simulink library "IPT_FCM_lib"  (Simulink 7.4)
settings: Solver=ode45  StartTime=0.0  StopTime=10.0  RelTol=1e-3
libraries: Defined_Functionality x62
settings Model: Creator=sunsijun  LastModifiedBy=sunsijun

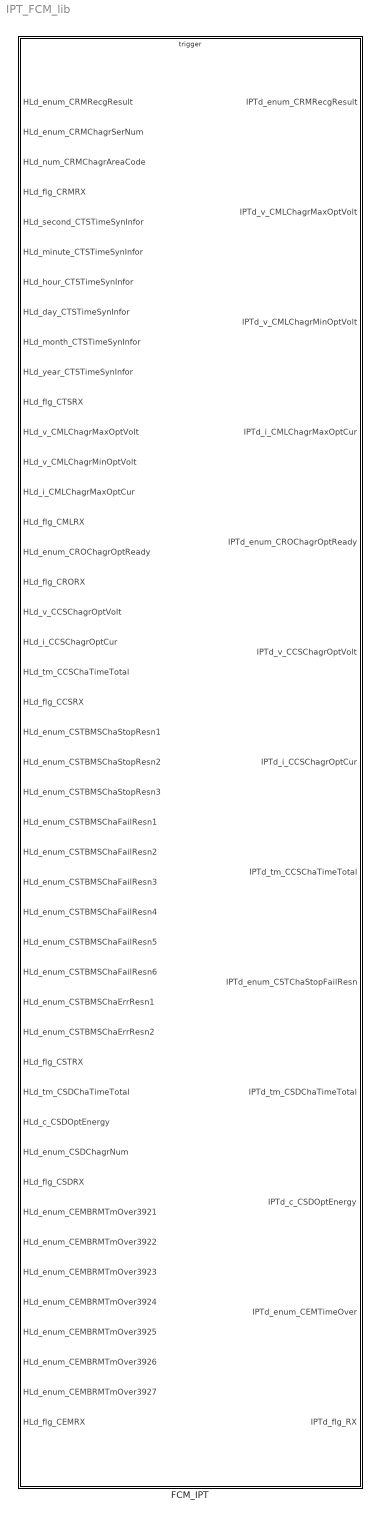
== system IPT_FCM_lib ==
  FCM_IPT : Subsystem  TreatAsAtomicUnit=on
      settings: RTWSystemCode=Function  RTWFcnNameOpts=Use subsystem name

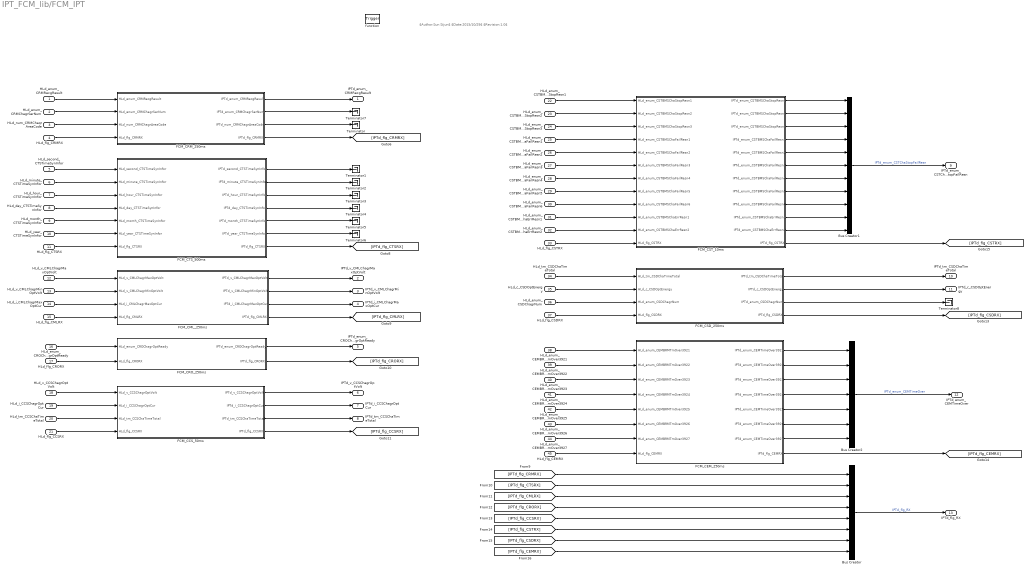
== system IPT_FCM_lib/FCM_IPT ==
  note: $Author:Sun Sijun$
      | $Date:2015/10/29$
      | $Revision:1.0$
  HLd_enum_CRMRecgResult : Inport
  HLd_enum_CRMChagrSerNum : Inport  Port=2
  HLd_num_CRMChagrAreaCode : Inport  Port=3
  HLd_flg_CRMRX : Inport  Port=4
  HLd_second_CTSTimeSynInfor : Inport  Port=5
  HLd_minute_CTSTimeSynInfor : Inport  Port=6
  HLd_hour_CTSTimeSynInfor : Inport  Port=7
  HLd_day_CTSTimeSynInfor : Inport  Port=8
  HLd_month_CTSTimeSynInfor : Inport  Port=9
  HLd_year_CTSTimeSynInfor : Inport  Port=10
  HLd_flg_CTSRX : Inport  Port=11
  HLd_v_CMLChagrMaxOptVolt : Inport  Port=12
  HLd_v_CMLChagrMinOptVolt : Inport  Port=13
  HLd_i_CMLChagrMaxOptCur : Inport  Port=14
  HLd_flg_CMLRX : Inport  Port=15
  HLd_enum_CROChagrOptReady : Inport  Port=16
  HLd_flg_CRORX : Inport  Port=17
  HLd_v_CCSChagrOptVolt : Inport  Port=18
  HLd_i_CCSChagrOptCur : Inport  Port=19
  HLd_tm_CCSChaTimeTotal : Inport  Port=20
  HLd_flg_CCSRX : Inport  Port=21
  HLd_enum_CSTBMSChaStopResn1 : Inport  Port=22
  HLd_enum_CSTBMSChaStopResn2 : Inport  Port=23
  HLd_enum_CSTBMSChaStopResn3 : Inport  Port=24
  HLd_enum_CSTBMSChaFailResn1 : Inport  Port=25
  HLd_enum_CSTBMSChaFailResn2 : Inport  Port=26
  HLd_enum_CSTBMSChaFailResn3 : Inport  Port=27
  HLd_enum_CSTBMSChaFailResn4 : Inport  Port=28
  HLd_enum_CSTBMSChaFailResn5 : Inport  Port=29
  HLd_enum_CSTBMSChaFailResn6 : Inport  Port=30
  HLd_enum_CSTBMSChaErrResn1 : Inport  Port=31
  HLd_enum_CSTBMSChaErrResn2 : Inport  Port=32
  HLd_flg_CSTRX : Inport  Port=33
  HLd_tm_CSDChaTimeTotal : Inport  Port=34
  HLd_c_CSDOptEnergy : Inport  Port=35
  HLd_enum_CSDChagrNum : Inport  Port=36
  HLd_flg_CSDRX : Inport  Port=37
  HLd_enum_CEMBRMTmOver3921 : Inport  Port=38
  HLd_enum_CEMBRMTmOver3922 : Inport  Port=39
  HLd_enum_CEMBRMTmOver3923 : Inport  Port=40
  HLd_enum_CEMBRMTmOver3924 : Inport  Port=41
  HLd_enum_CEMBRMTmOver3925 : Inport  Port=42
  HLd_enum_CEMBRMTmOver3926 : Inport  Port=43
  HLd_enum_CEMBRMTmOver3927 : Inport  Port=44
  HLd_flg_CEMRX : Inport  Port=45
  function : TriggerPort  TriggerType=function-call
  Bus Creator : BusCreator  Inputs=8
  Bus Creator1 : BusCreator  Inputs=11
  Bus Creator2 : BusCreator  Inputs=7
  FCM_CCS_50ms : Subsystem
      settings: RTWFcnNameOpts=Use subsystem name  RTWFileNameOpts=Use subsystem name
  FCM_CEM_250ms : Subsystem
      settings: RTWFcnNameOpts=Use subsystem name  RTWFileNameOpts=Use subsystem name
  FCM_CML_250ms : Subsystem
      settings: RTWFcnNameOpts=Use subsystem name  RTWFileNameOpts=Use subsystem name
  FCM_CRM_250ms : Subsystem
      settings: RTWFcnNameOpts=Use subsystem name  RTWFileNameOpts=Use subsystem name
  FCM_CRO_250ms : Subsystem
      settings: RTWFcnNameOpts=Use subsystem name  RTWFileNameOpts=Use subsystem name
  FCM_CSD_250ms : Subsystem
      settings: RTWFcnNameOpts=Use subsystem name  RTWFileNameOpts=Use subsystem name
  FCM_CST_10ms : Subsystem
      settings: RTWFcnNameOpts=Use subsystem name  RTWFileNameOpts=Use subsystem name
  FCM_CTS_500ms : Subsystem
      settings: RTWFcnNameOpts=Use subsystem name  RTWFileNameOpts=Use subsystem name
  Terminator{,1..8} (9 alike) : Terminator
  IPTd_enum_CRMRecgResult : Outport
  IPTd_v_CMLChagrMaxOptVolt : Outport  Port=2
  IPTd_v_CMLChagrMinOptVolt : Outport  Port=3
  IPTd_i_CMLChagrMaxOptCur : Outport  Port=4
  IPTd_enum_CROChagrOptReady : Outport  Port=5
  IPTd_v_CCSChagrOptVolt : Outport  Port=6
  IPTd_i_CCSChagrOptCur : Outport  Port=7
  IPTd_tm_CCSChaTimeTotal : Outport  Port=8
  IPTd_enum_CSTChaStopFailResn : Outport  Port=9
  IPTd_tm_CSDChaTimeTotal : Outport  Port=10
  IPTd_c_CSDOptEnergy : Outport  Port=11
  IPTd_enum_CEMTimeOver : Outport  Port=12
  IPTd_flg_RX : Outport  Port=13
  wires:
  HLd_flg_CEMRX/1 -> FCM_CEM_250ms/8(HLd_flg_CEMRX)
  HLd_flg_CSDRX/1 -> FCM_CSD_250ms/4(HLd_flg_CSDRX)
  HLd_flg_CSTRX/1 -> FCM_CST_10ms/12(HLd_flg_CSTRX)
  HLd_flg_CCSRX/1 -> FCM_CCS_50ms/4(HLd_flg_CCSRX)
  HLd_flg_CRORX/1 -> FCM_CRO_250ms/2(HLd_flg_CRORX)
  HLd_flg_CMLRX/1 -> FCM_CML_250ms/4(HLd_flg_CMLRX)
  HLd_flg_CTSRX/1 -> FCM_CTS_500ms/7(HLd_flg_CTSRX)
  HLd_flg_CRMRX/1 -> FCM_CRM_250ms/4(HLd_flg_CRMRX)
  Bus Creator1/1 -> IPTd_enum_CSTChaStopFailResn/1  "IPTd_enum_CSTChaStopFailResn"
  Bus Creator2/1 -> IPTd_enum_CEMTimeOver/1  "IPTd_enum_CEMTimeOver"
  FCM_CST_10ms/11(IPTd_enum_CSTBMSChaErrResn2) -> Bus Creator1/11
  FCM_CST_10ms/10(IPTd_enum_CSTBMSChaErrResn1) -> Bus Creator1/10
  FCM_CST_10ms/9(IPTd_enum_CSTBMSChaFailResn6) -> Bus Creator1/9
  FCM_CST_10ms/8(IPTd_enum_CSTBMSChaFailResn5) -> Bus Creator1/8
  FCM_CST_10ms/7(IPTd_enum_CSTBMSChaFailResn4) -> Bus Creator1/7
  FCM_CST_10ms/6(IPTd_enum_CSTBMSChaFailResn3) -> Bus Creator1/6
  FCM_CST_10ms/5(IPTd_enum_CSTBMSChaFailResn2) -> Bus Creator1/5
  FCM_CST_10ms/4(IPTd_enum_CSTBMSChaFailResn1) -> Bus Creator1/4
  FCM_CST_10ms/3(IPTd_enum_CSTBMSChaStopResn3) -> Bus Creator1/3
  FCM_CST_10ms/2(IPTd_enum_CSTBMSChaStopResn2) -> Bus Creator1/2
  FCM_CST_10ms/1(IPTd_enum_CSTBMSChaStopResn1) -> Bus Creator1/1
  Bus Creator/1 -> IPTd_flg_RX/1  "IPTd_flg_RX"
  [IPTd_flg_CEMRX] -> Bus Creator/8
  [IPTd_flg_CSDRX] -> Bus Creator/7
  [IPTd_flg_CSTRX] -> Bus Creator/6
  [IPTd_flg_CCSRX] -> Bus Creator/5
  [IPTd_flg_CRORX] -> Bus Creator/4
  [IPTd_flg_CMLRX] -> Bus Creator/3
  [IPTd_flg_CTSRX] -> Bus Creator/2
  [IPTd_flg_CRMRX] -> Bus Creator/1
  FCM_CEM_250ms/8(IPTd_flg_CEMRX) -> [IPTd_flg_CEMRX]
  FCM_CSD_250ms/4(IPTd_flg_CSDRX) -> [IPTd_flg_CSDRX]
  FCM_CST_10ms/12(IPTd_flg_CSTRX) -> [IPTd_flg_CSTRX]
  FCM_CCS_50ms/4(IPTd_flg_CCSRX) -> [IPTd_flg_CCSRX]
  FCM_CRO_250ms/2(IPTd_flg_CRORX) -> [IPTd_flg_CRORX]
  FCM_CEM_250ms/1(IPTd_enum_CEMTimeOver3921) -> Bus Creator2/1
  FCM_CEM_250ms/2(IPTd_enum_CEMTimeOver3922) -> Bus Creator2/2
  FCM_CEM_250ms/3(IPTd_enum_CEMTimeOver3923) -> Bus Creator2/3
  FCM_CEM_250ms/4(IPTd_enum_CEMTimeOver3924) -> Bus Creator2/4
  FCM_CEM_250ms/5(IPTd_enum_CEMTimeOver3925) -> Bus Creator2/5
  FCM_CEM_250ms/6(IPTd_enum_CEMTimeOver3926) -> Bus Creator2/6
  FCM_CEM_250ms/7(IPTd_enum_CEMTimeOver3927) -> Bus Creator2/7
  HLd_enum_CEMBRMTmOver3921/1 -> FCM_CEM_250ms/1(HLd_enum_CEMBRMTmOver3921)
  HLd_enum_CEMBRMTmOver3922/1 -> FCM_CEM_250ms/2(HLd_enum_CEMBRMTmOver3922)
  HLd_enum_CEMBRMTmOver3923/1 -> FCM_CEM_250ms/3(HLd_enum_CEMBRMTmOver3923)
  HLd_enum_CEMBRMTmOver3924/1 -> FCM_CEM_250ms/4(HLd_enum_CEMBRMTmOver3924)
  HLd_enum_CEMBRMTmOver3925/1 -> FCM_CEM_250ms/5(HLd_enum_CEMBRMTmOver3925)
  HLd_enum_CEMBRMTmOver3926/1 -> FCM_CEM_250ms/6(HLd_enum_CEMBRMTmOver3926)
  HLd_enum_CEMBRMTmOver3927/1 -> FCM_CEM_250ms/7(HLd_enum_CEMBRMTmOver3927)
  HLd_tm_CSDChaTimeTotal/1 -> FCM_CSD_250ms/1(HLd_tm_CSDChaTimeTotal)
  HLd_c_CSDOptEnergy/1 -> FCM_CSD_250ms/2(HLd_c_CSDOptEnergy)
  HLd_enum_CSDChagrNum/1 -> FCM_CSD_250ms/3(HLd_enum_CSDChagrNum)
  FCM_CSD_250ms/3(IPTd_enum_CSDChagrNum) -> Terminator8/1
  FCM_CSD_250ms/2(IPTd_c_CSDOptEnergy) -> IPTd_c_CSDOptEnergy/1
  FCM_CSD_250ms/1(IPTd_tm_CSDChaTimeTotal) -> IPTd_tm_CSDChaTimeTotal/1
  HLd_enum_CSTBMSChaErrResn2/1 -> FCM_CST_10ms/11(HLd_enum_CSTBMSChaErrResn2)
  HLd_enum_CSTBMSChaErrResn1/1 -> FCM_CST_10ms/10(HLd_enum_CSTBMSChaErrResn1)
  HLd_enum_CSTBMSChaFailResn6/1 -> FCM_CST_10ms/9(HLd_enum_CSTBMSChaFailResn6)
  HLd_enum_CSTBMSChaFailResn5/1 -> FCM_CST_10ms/8(HLd_enum_CSTBMSChaFailResn5)
  HLd_enum_CSTBMSChaFailResn4/1 -> FCM_CST_10ms/7(HLd_enum_CSTBMSChaFailResn4)
  HLd_enum_CSTBMSChaFailResn3/1 -> FCM_CST_10ms/6(HLd_enum_CSTBMSChaFailResn3)
  HLd_enum_CSTBMSChaFailResn2/1 -> FCM_CST_10ms/5(HLd_enum_CSTBMSChaFailResn2)
  HLd_enum_CSTBMSChaFailResn1/1 -> FCM_CST_10ms/4(HLd_enum_CSTBMSChaFailResn1)
  HLd_enum_CSTBMSChaStopResn3/1 -> FCM_CST_10ms/3(HLd_enum_CSTBMSChaStopResn3)
  HLd_enum_CSTBMSChaStopResn2/1 -> FCM_CST_10ms/2(HLd_enum_CSTBMSChaStopResn2)
  HLd_enum_CSTBMSChaStopResn1/1 -> FCM_CST_10ms/1(HLd_enum_CSTBMSChaStopResn1)
  FCM_CCS_50ms/3(IPTd_tm_CCSChaTimeTotal) -> IPTd_tm_CCSChaTimeTotal/1
  FCM_CCS_50ms/2(IPTd_i_CCSChagrOptCur) -> IPTd_i_CCSChagrOptCur/1
  FCM_CCS_50ms/1(IPTd_v_CCSChagrOptVolt) -> IPTd_v_CCSChagrOptVolt/1
  HLd_tm_CCSChaTimeTotal/1 -> FCM_CCS_50ms/3(HLd_tm_CCSChaTimeTotal)
  HLd_i_CCSChagrOptCur/1 -> FCM_CCS_50ms/2(HLd_i_CCSChagrOptCur)
  HLd_v_CCSChagrOptVolt/1 -> FCM_CCS_50ms/1(HLd_v_CCSChagrOptVolt)
  HLd_enum_CROChagrOptReady/1 -> FCM_CRO_250ms/1(HLd_enum_CROChagrOptReady)
  FCM_CRO_250ms/1(IPTd_enum_CROChagrOptReady) -> IPTd_enum_CROChagrOptReady/1
  FCM_CML_250ms/1(IPTd_v_CMLChagrMaxOptVolt) -> IPTd_v_CMLChagrMaxOptVolt/1
  FCM_CML_250ms/2(IPTd_v_CMLChagrMinOptVolt) -> IPTd_v_CMLChagrMinOptVolt/1
  FCM_CML_250ms/3(IPTd_i_CMLChagrMaxOptCur) -> IPTd_i_CMLChagrMaxOptCur/1
  HLd_v_CMLChagrMaxOptVolt/1 -> FCM_CML_250ms/1(HLd_v_CMLChagrMaxOptVolt)
  HLd_v_CMLChagrMinOptVolt/1 -> FCM_CML_250ms/2(HLd_v_CMLChagrMinOptVolt)
  HLd_i_CMLChagrMaxOptCur/1 -> FCM_CML_250ms/3(HLd_i_CMLChagrMaxOptCur)
  HLd_year_CTSTimeSynInfor/1 -> FCM_CTS_500ms/6(HLd_year_CTSTimeSynInfor)
  HLd_month_CTSTimeSynInfor/1 -> FCM_CTS_500ms/5(HLd_month_CTSTimeSynInfor)
  HLd_day_CTSTimeSynInfor/1 -> FCM_CTS_500ms/4(HLd_day_CTSTimeSynInfor)
  HLd_hour_CTSTimeSynInfor/1 -> FCM_CTS_500ms/3(HLd_hour_CTSTimeSynInfor)
  HLd_minute_CTSTimeSynInfor/1 -> FCM_CTS_500ms/2(HLd_minute_CTSTimeSynInfor)
  HLd_second_CTSTimeSynInfor/1 -> FCM_CTS_500ms/1(HLd_second_CTSTimeSynInfor)
  FCM_CRM_250ms/3(IPTd_num_CRMChagrAreaCode) -> Terminator/1
  FCM_CRM_250ms/2(IPTd_enum_CRMChagrSerNum) -> Terminator7/1
  FCM_CRM_250ms/1(IPTd_enum_CRMRecgResult) -> IPTd_enum_CRMRecgResult/1
  HLd_num_CRMChagrAreaCode/1 -> FCM_CRM_250ms/3(HLd_num_CRMChagrAreaCode)
  HLd_enum_CRMChagrSerNum/1 -> FCM_CRM_250ms/2(HLd_enum_CRMChagrSerNum)
  HLd_enum_CRMRecgResult/1 -> FCM_CRM_250ms/1(HLd_enum_CRMRecgResult)
  FCM_CML_250ms/4(IPTd_flg_CMLRX) -> [IPTd_flg_CMLRX]
  FCM_CTS_500ms/6(IPTd_year_CTSTimeSynInfor) -> Terminator6/1
  FCM_CTS_500ms/5(IPTd_month_CTSTimeSynInfor) -> Terminator5/1
  FCM_CTS_500ms/4(IPTd_day_CTSTimeSynInfor) -> Terminator4/1
  FCM_CTS_500ms/3(IPTd_hour_CTSTimeSynInfor) -> Terminator3/1
  FCM_CTS_500ms/2(IPTd_minute_CTSTimeSynInfor) -> Terminator2/1
  FCM_CTS_500ms/1(IPTd_second_CTSTimeSynInfor) -> Terminator1/1
  FCM_CTS_500ms/7(IPTd_flg_CTSRX) -> [IPTd_flg_CTSRX]
  FCM_CRM_250ms/4(IPTd_flg_CRMRX) -> [IPTd_flg_CRMRX]

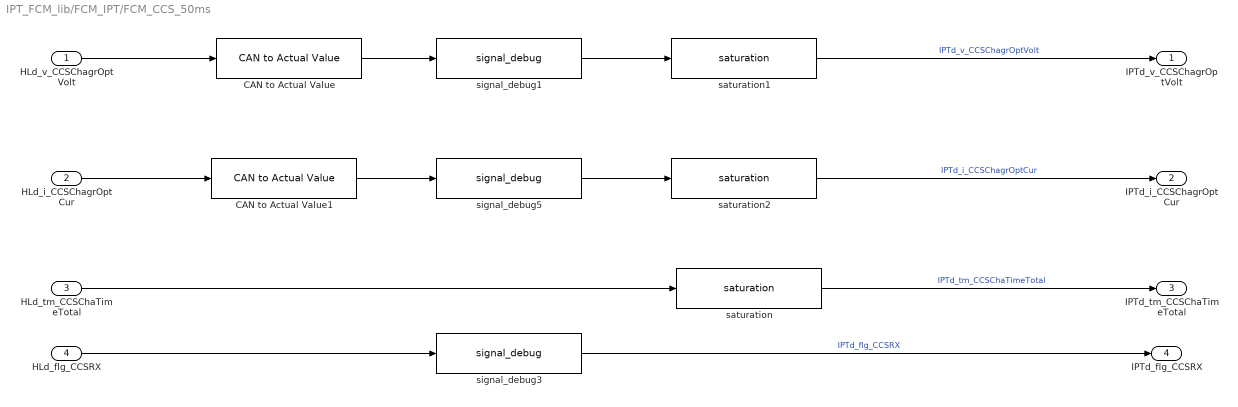
== system IPT_FCM_lib/FCM_IPT/FCM_CCS_50ms ==
  HLd_v_CCSChagrOptVolt : Inport
  HLd_i_CCSChagrOptCur : Inport  Port=2
  HLd_tm_CCSChaTimeTotal : Inport  Port=3
  HLd_flg_CCSRX : Inport  Port=4
  CAN to Actual Value : Defined_Functionality/CAN to Actual Value  SystemSampleTime=-1  gain=0.1  offset=0
      settings: AttributesFormatString=[GAIN=%<gain>]\n[OFFSET=%<offset>]
  CAN to Actual Value1 : Defined_Functionality/CAN to Actual Value  SystemSampleTime=-1  gain=0.1  offset=-400
      settings: AttributesFormatString=[GAIN=%<gain>]\n[OFFSET=%<offset>]
  saturation : Defined_Functionality/saturation  SystemSampleTime=-1  upper_limit=600  lower_limit=0
      settings: AttributesFormatString=[UPPER_LIMIT=%<upper_limit>]\n[LOWER_LIMIT=%<lower_limit>]
  saturation1 : Defined_Functionality/saturation  SystemSampleTime=-1  upper_limit=750  lower_limit=0
      settings: AttributesFormatString=[UPPER_LIMIT=%<upper_limit>]\n[LOWER_LIMIT=%<lower_limit>]
  saturation2 : Defined_Functionality/saturation  SystemSampleTime=-1  upper_limit=0  lower_limit=-400
      settings: AttributesFormatString=[UPPER_LIMIT=%<upper_limit>]\n[LOWER_LIMIT=%<lower_limit>]
  signal_debug1 : Defined_Functionality/signal_debug  SystemSampleTime=-1  debug_switch=IPTc_dbgsw_CCSChagrOptVolt  debug_value=IPTc_dbgval_CCSChagrOptVolt
      settings: AttributesFormatString=[SWITCH=%<debug_switch>]\n[VALUE=%<debug_value>]
  signal_debug3 : Defined_Functionality/signal_debug  SystemSampleTime=-1  debug_switch=IPTc_dbgsw_CCSRX  debug_value=IPTc_dbgval_CCSRX
      settings: AttributesFormatString=[SWITCH=%<debug_switch>]\n[VALUE=%<debug_value>]
  signal_debug5 : Defined_Functionality/signal_debug  SystemSampleTime=-1  debug_switch=IPTc_dbgsw_CCSChagrOptCur  debug_value=IPTc_dbgval_CCSChagrOptCur
      settings: AttributesFormatString=[SWITCH=%<debug_switch>]\n[VALUE=%<debug_value>]
  IPTd_v_CCSChagrOptVolt : Outport
  IPTd_i_CCSChagrOptCur : Outport  Port=2
  IPTd_tm_CCSChaTimeTotal : Outport  Port=3
  IPTd_flg_CCSRX : Outport  Port=4
  wires:
  HLd_flg_CCSRX/1 -> signal_debug3/1
  signal_debug3/1 -> IPTd_flg_CCSRX/1  "IPTd_flg_CCSRX"
  saturation2/1 -> IPTd_i_CCSChagrOptCur/1  "IPTd_i_CCSChagrOptCur"
  saturation1/1 -> IPTd_v_CCSChagrOptVolt/1  "IPTd_v_CCSChagrOptVolt"
  HLd_i_CCSChagrOptCur/1 -> CAN to Actual Value1/1
  HLd_v_CCSChagrOptVolt/1 -> CAN to Actual Value/1
  signal_debug1/1 -> saturation1/1
  CAN to Actual Value1/1 -> signal_debug5/1
  CAN to Actual Value/1 -> signal_debug1/1
  signal_debug5/1 -> saturation2/1
  saturation/1 -> IPTd_tm_CCSChaTimeTotal/1  "IPTd_tm_CCSChaTimeTotal"
  HLd_tm_CCSChaTimeTotal/1 -> saturation/1

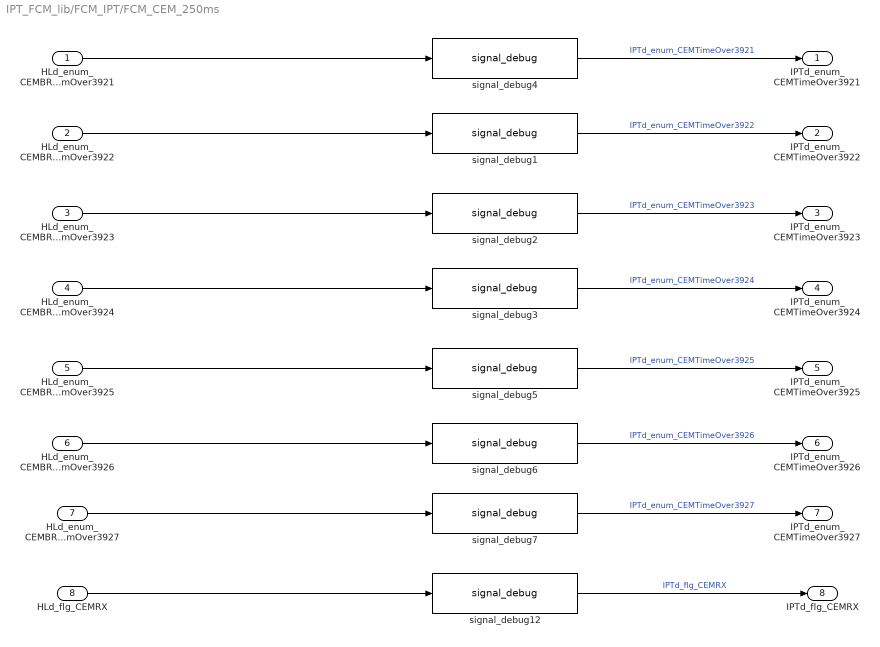
== system IPT_FCM_lib/FCM_IPT/FCM_CEM_250ms ==
  HLd_enum_CEMBRMTmOver3921 : Inport
  HLd_enum_CEMBRMTmOver3922 : Inport  Port=2
  HLd_enum_CEMBRMTmOver3923 : Inport  Port=3
  HLd_enum_CEMBRMTmOver3924 : Inport  Port=4
  HLd_enum_CEMBRMTmOver3925 : Inport  Port=5
  HLd_enum_CEMBRMTmOver3926 : Inport  Port=6
  HLd_enum_CEMBRMTmOver3927 : Inport  Port=7
  HLd_flg_CEMRX : Inport  Port=8
  signal_debug1 : Defined_Functionality/signal_debug  SystemSampleTime=-1  debug_switch=IPTc_dbgsw_CEMBRMTmOver3922  debug_value=IPTc_dbgval_CEMBRMTmOver3922
      settings: AttributesFormatString=[SWITCH=%<debug_switch>]\n[VALUE=%<debug_value>]
  signal_debug12 : Defined_Functionality/signal_debug  SystemSampleTime=-1  debug_switch=IPTc_dbgsw_CSDRX  debug_value=IPTc_dbgval_CSDRX
      settings: AttributesFormatString=[SWITCH=%<debug_switch>]\n[VALUE=%<debug_value>]
  signal_debug2 : Defined_Functionality/signal_debug  SystemSampleTime=-1  debug_switch=IPTc_dbgsw_CEMBRMTmOver3923  debug_value=IPTc_dbgval_CEMBRMTmOver3923
      settings: AttributesFormatString=[SWITCH=%<debug_switch>]\n[VALUE=%<debug_value>]
  signal_debug3 : Defined_Functionality/signal_debug  SystemSampleTime=-1  debug_switch=IPTc_dbgsw_CEMBRMTmOver3924  debug_value=IPTc_dbgval_CEMBRMTmOver3924
      settings: AttributesFormatString=[SWITCH=%<debug_switch>]\n[VALUE=%<debug_value>]
  signal_debug4 : Defined_Functionality/signal_debug  SystemSampleTime=-1  debug_switch=IPTc_dbgsw_CEMBRMTmOver3921  debug_value=IPTc_dbgval_CEMBRMTmOver3921
      settings: AttributesFormatString=[SWITCH=%<debug_switch>]\n[VALUE=%<debug_value>]
  signal_debug5 : Defined_Functionality/signal_debug  SystemSampleTime=-1  debug_switch=IPTc_dbgsw_CEMBRMTmOver3925  debug_value=IPTc_dbgval_CEMBRMTmOver3925
      settings: AttributesFormatString=[SWITCH=%<debug_switch>]\n[VALUE=%<debug_value>]
  signal_debug6 : Defined_Functionality/signal_debug  SystemSampleTime=-1  debug_switch=IPTc_dbgsw_CEMBRMTmOver3926  debug_value=IPTc_dbgval_CEMBRMTmOver3926
      settings: AttributesFormatString=[SWITCH=%<debug_switch>]\n[VALUE=%<debug_value>]
  signal_debug7 : Defined_Functionality/signal_debug  SystemSampleTime=-1  debug_switch=IPTc_dbgsw_CEMBRMTmOver3927  debug_value=IPTc_dbgval_CEMBRMTmOver3927
      settings: AttributesFormatString=[SWITCH=%<debug_switch>]\n[VALUE=%<debug_value>]
  IPTd_enum_CEMTimeOver3921 : Outport
  IPTd_enum_CEMTimeOver3922 : Outport  Port=2
  IPTd_enum_CEMTimeOver3923 : Outport  Port=3
  IPTd_enum_CEMTimeOver3924 : Outport  Port=4
  IPTd_enum_CEMTimeOver3925 : Outport  Port=5
  IPTd_enum_CEMTimeOver3926 : Outport  Port=6
  IPTd_enum_CEMTimeOver3927 : Outport  Port=7
  IPTd_flg_CEMRX : Outport  Port=8
  wires:
  signal_debug12/1 -> IPTd_flg_CEMRX/1  "IPTd_flg_CEMRX"
  HLd_flg_CEMRX/1 -> signal_debug12/1
  signal_debug5/1 -> IPTd_enum_CEMTimeOver3925/1  "IPTd_enum_CEMTimeOver3925"
  signal_debug7/1 -> IPTd_enum_CEMTimeOver3927/1  "IPTd_enum_CEMTimeOver3927"
  signal_debug6/1 -> IPTd_enum_CEMTimeOver3926/1  "IPTd_enum_CEMTimeOver3926"
  HLd_enum_CEMBRMTmOver3927/1 -> signal_debug7/1
  HLd_enum_CEMBRMTmOver3926/1 -> signal_debug6/1
  HLd_enum_CEMBRMTmOver3925/1 -> signal_debug5/1
  HLd_enum_CEMBRMTmOver3924/1 -> signal_debug3/1
  signal_debug3/1 -> IPTd_enum_CEMTimeOver3924/1  "IPTd_enum_CEMTimeOver3924"
  signal_debug2/1 -> IPTd_enum_CEMTimeOver3923/1  "IPTd_enum_CEMTimeOver3923"
  HLd_enum_CEMBRMTmOver3923/1 -> signal_debug2/1
  signal_debug1/1 -> IPTd_enum_CEMTimeOver3922/1  "IPTd_enum_CEMTimeOver3922"
  HLd_enum_CEMBRMTmOver3922/1 -> signal_debug1/1
  signal_debug4/1 -> IPTd_enum_CEMTimeOver3921/1  "IPTd_enum_CEMTimeOver3921"
  HLd_enum_CEMBRMTmOver3921/1 -> signal_debug4/1

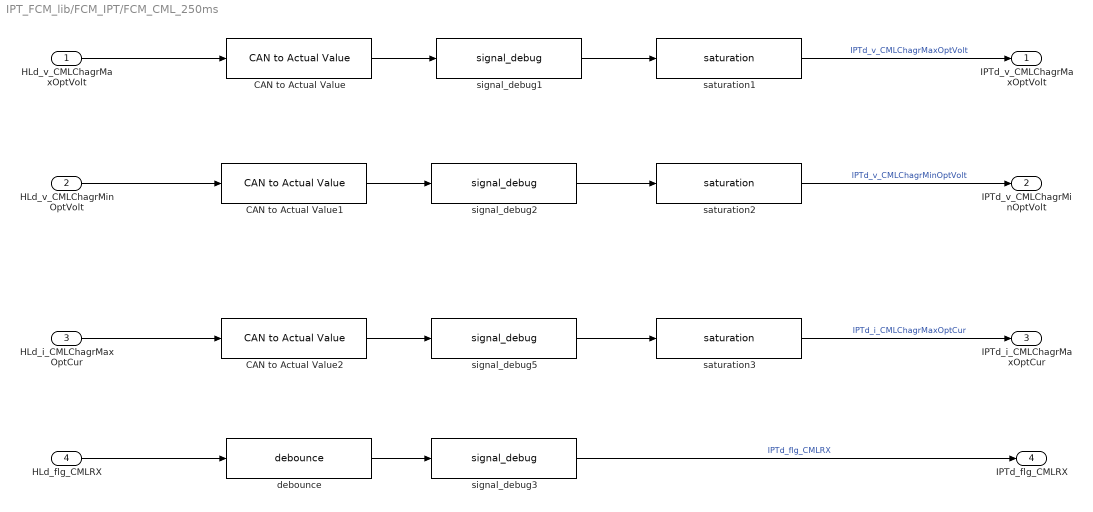
== system IPT_FCM_lib/FCM_IPT/FCM_CML_250ms ==
  HLd_v_CMLChagrMaxOptVolt : Inport
  HLd_v_CMLChagrMinOptVolt : Inport  Port=2
  HLd_i_CMLChagrMaxOptCur : Inport  Port=3
  HLd_flg_CMLRX : Inport  Port=4
  CAN to Actual Value : Defined_Functionality/CAN to Actual Value  SystemSampleTime=-1  gain=0.1  offset=0
      settings: AttributesFormatString=[GAIN=%<gain>]\n[OFFSET=%<offset>]
  CAN to Actual Value1 : Defined_Functionality/CAN to Actual Value  SystemSampleTime=-1  gain=0.1  offset=0
      settings: AttributesFormatString=[GAIN=%<gain>]\n[OFFSET=%<offset>]
  CAN to Actual Value2 : Defined_Functionality/CAN to Actual Value  SystemSampleTime=-1  gain=0.1  offset=-400
      settings: AttributesFormatString=[GAIN=%<gain>]\n[OFFSET=%<offset>]
  debounce : Defined_Functionality/debounce  SystemSampleTime=-1  debounce_time=30
      settings: AttributesFormatString=[DEBOUNCE_TIME=%<debounce_time>]
  saturation1 : Defined_Functionality/saturation  SystemSampleTime=-1  upper_limit=750  lower_limit=0
      settings: AttributesFormatString=[UPPER_LIMIT=%<upper_limit>]\n[LOWER_LIMIT=%<lower_limit>]
  saturation2 : Defined_Functionality/saturation  SystemSampleTime=-1  upper_limit=750  lower_limit=0
      settings: AttributesFormatString=[UPPER_LIMIT=%<upper_limit>]\n[LOWER_LIMIT=%<lower_limit>]
  saturation3 : Defined_Functionality/saturation  SystemSampleTime=-1  upper_limit=0  lower_limit=-400
      settings: AttributesFormatString=[UPPER_LIMIT=%<upper_limit>]\n[LOWER_LIMIT=%<lower_limit>]
  signal_debug1 : Defined_Functionality/signal_debug  SystemSampleTime=-1  debug_switch=IPTc_dbgsw_CMLChagrMaxOptVolt  debug_value=IPTc_dbgval_CMLChagrMaxOptVolt
      settings: AttributesFormatString=[SWITCH=%<debug_switch>]\n[VALUE=%<debug_value>]
  signal_debug2 : Defined_Functionality/signal_debug  SystemSampleTime=-1  debug_switch=IPTc_dbgsw_CMLChagrMinOptVolt  debug_value=IPTc_dbgval_CMLChagrMinOptVolt
      settings: AttributesFormatString=[SWITCH=%<debug_switch>]\n[VALUE=%<debug_value>]
  signal_debug3 : Defined_Functionality/signal_debug  SystemSampleTime=-1  debug_switch=IPTc_dbgsw_CMLRX  debug_value=IPTc_dbgval_CMLRX
      settings: AttributesFormatString=[SWITCH=%<debug_switch>]\n[VALUE=%<debug_value>]
  signal_debug5 : Defined_Functionality/signal_debug  SystemSampleTime=-1  debug_switch=IPTc_dbgsw_CMLChagrMaxOptCur  debug_value=IPTc_dbgval_CMLChagrMaxOptCur
      settings: AttributesFormatString=[SWITCH=%<debug_switch>]\n[VALUE=%<debug_value>]
  IPTd_v_CMLChagrMaxOptVolt : Outport
  IPTd_v_CMLChagrMinOptVolt : Outport  Port=2
  IPTd_i_CMLChagrMaxOptCur : Outport  Port=3
  IPTd_flg_CMLRX : Outport  Port=4
  wires:
  debounce/1 -> signal_debug3/1
  HLd_flg_CMLRX/1 -> debounce/1
  signal_debug3/1 -> IPTd_flg_CMLRX/1  "IPTd_flg_CMLRX"
  saturation3/1 -> IPTd_i_CMLChagrMaxOptCur/1  "IPTd_i_CMLChagrMaxOptCur"
  saturation2/1 -> IPTd_v_CMLChagrMinOptVolt/1  "IPTd_v_CMLChagrMinOptVolt"
  signal_debug1/1 -> saturation1/1
  saturation1/1 -> IPTd_v_CMLChagrMaxOptVolt/1  "IPTd_v_CMLChagrMaxOptVolt"
  HLd_i_CMLChagrMaxOptCur/1 -> CAN to Actual Value2/1
  HLd_v_CMLChagrMinOptVolt/1 -> CAN to Actual Value1/1
  HLd_v_CMLChagrMaxOptVolt/1 -> CAN to Actual Value/1
  signal_debug5/1 -> saturation3/1
  CAN to Actual Value2/1 -> signal_debug5/1
  CAN to Actual Value1/1 -> signal_debug2/1
  signal_debug2/1 -> saturation2/1
  CAN to Actual Value/1 -> signal_debug1/1

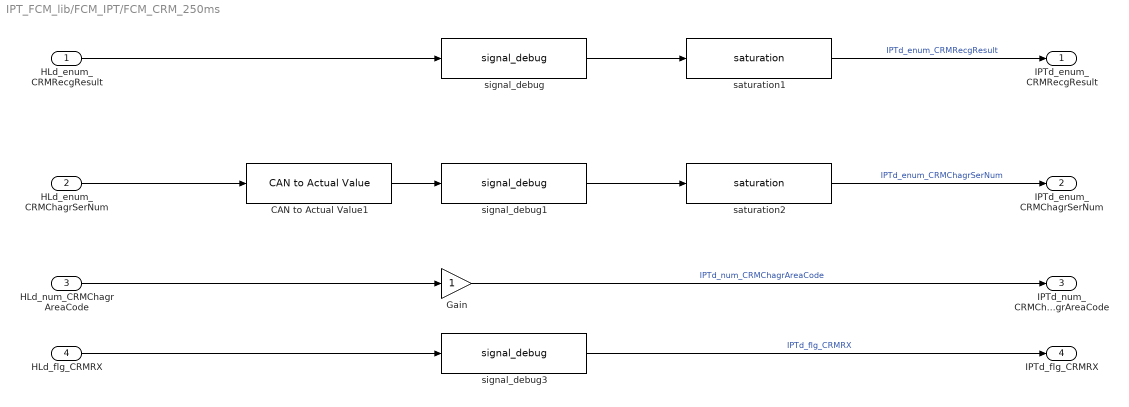
== system IPT_FCM_lib/FCM_IPT/FCM_CRM_250ms ==
  HLd_enum_CRMRecgResult : Inport
  HLd_enum_CRMChagrSerNum : Inport  Port=2
  HLd_num_CRMChagrAreaCode : Inport  Port=3
  HLd_flg_CRMRX : Inport  Port=4
  CAN to Actual Value1 : Defined_Functionality/CAN to Actual Value  SystemSampleTime=-1  gain=1  offset=1
      settings: AttributesFormatString=[GAIN=%<gain>]\n[OFFSET=%<offset>]
  Gain : Gain  OutDataTypeStr=Inherit: Same as input
  saturation1 : Defined_Functionality/saturation  SystemSampleTime=-1  upper_limit=255  lower_limit=0
      settings: AttributesFormatString=[UPPER_LIMIT=%<upper_limit>]\n[LOWER_LIMIT=%<lower_limit>]
  saturation2 : Defined_Functionality/saturation  SystemSampleTime=-1  upper_limit=100  lower_limit=1
      settings: AttributesFormatString=[UPPER_LIMIT=%<upper_limit>]\n[LOWER_LIMIT=%<lower_limit>]
  signal_debug : Defined_Functionality/signal_debug  SystemSampleTime=-1  debug_switch=IPTc_dbgsw_CRMRecgResult  debug_value=IPTc_dbgval_CRMRecgResult
      settings: AttributesFormatString=[SWITCH=%<debug_switch>]\n[VALUE=%<debug_value>]
  signal_debug1 : Defined_Functionality/signal_debug  SystemSampleTime=-1  debug_switch=IPTc_dbgsw_CRMChagrSerNum  debug_value=IPTc_dbgval_CRMChagrSerNum
      settings: AttributesFormatString=[SWITCH=%<debug_switch>]\n[VALUE=%<debug_value>]
  signal_debug3 : Defined_Functionality/signal_debug  SystemSampleTime=-1  debug_switch=IPTc_dbgsw_CRMRX  debug_value=IPTc_dbgval_CRMRX
      settings: AttributesFormatString=[SWITCH=%<debug_switch>]\n[VALUE=%<debug_value>]
  IPTd_enum_CRMRecgResult : Outport
  IPTd_enum_CRMChagrSerNum : Outport  Port=2
  IPTd_num_CRMChagrAreaCode : Outport  Port=3
  IPTd_flg_CRMRX : Outport  Port=4
  wires:
  signal_debug3/1 -> IPTd_flg_CRMRX/1  "IPTd_flg_CRMRX"
  HLd_flg_CRMRX/1 -> signal_debug3/1
  saturation2/1 -> IPTd_enum_CRMChagrSerNum/1  "IPTd_enum_CRMChagrSerNum"
  saturation1/1 -> IPTd_enum_CRMRecgResult/1  "IPTd_enum_CRMRecgResult"
  Gain/1 -> IPTd_num_CRMChagrAreaCode/1  "IPTd_num_CRMChagrAreaCode"
  CAN to Actual Value1/1 -> signal_debug1/1
  signal_debug1/1 -> saturation2/1
  signal_debug/1 -> saturation1/1
  HLd_enum_CRMRecgResult/1 -> signal_debug/1
  HLd_num_CRMChagrAreaCode/1 -> Gain/1
  HLd_enum_CRMChagrSerNum/1 -> CAN to Actual Value1/1

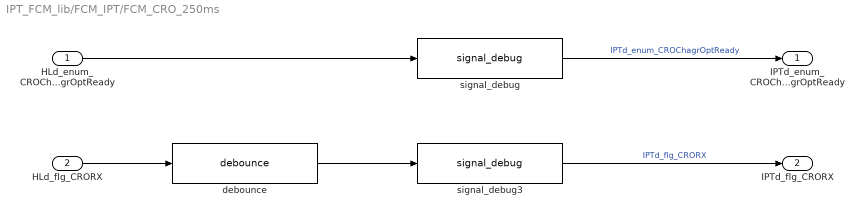
== system IPT_FCM_lib/FCM_IPT/FCM_CRO_250ms ==
  HLd_enum_CROChagrOptReady : Inport
  HLd_flg_CRORX : Inport  Port=2
  debounce : Defined_Functionality/debounce  SystemSampleTime=-1  debounce_time=30
      settings: AttributesFormatString=[DEBOUNCE_TIME=%<debounce_time>]
  signal_debug : Defined_Functionality/signal_debug  SystemSampleTime=-1  debug_switch=IPTc_dbgsw_CROChagrOptReady  debug_value=IPTc_dbgval_CROChagrOptReady
      settings: AttributesFormatString=[SWITCH=%<debug_switch>]\n[VALUE=%<debug_value>]
  signal_debug3 : Defined_Functionality/signal_debug  SystemSampleTime=-1  debug_switch=IPTc_dbgsw_CRORX  debug_value=IPTc_dbgval_CRORX
      settings: AttributesFormatString=[SWITCH=%<debug_switch>]\n[VALUE=%<debug_value>]
  IPTd_enum_CROChagrOptReady : Outport
  IPTd_flg_CRORX : Outport  Port=2
  wires:
  debounce/1 -> signal_debug3/1
  HLd_flg_CRORX/1 -> debounce/1
  signal_debug3/1 -> IPTd_flg_CRORX/1  "IPTd_flg_CRORX"
  signal_debug/1 -> IPTd_enum_CROChagrOptReady/1  "IPTd_enum_CROChagrOptReady"
  HLd_enum_CROChagrOptReady/1 -> signal_debug/1

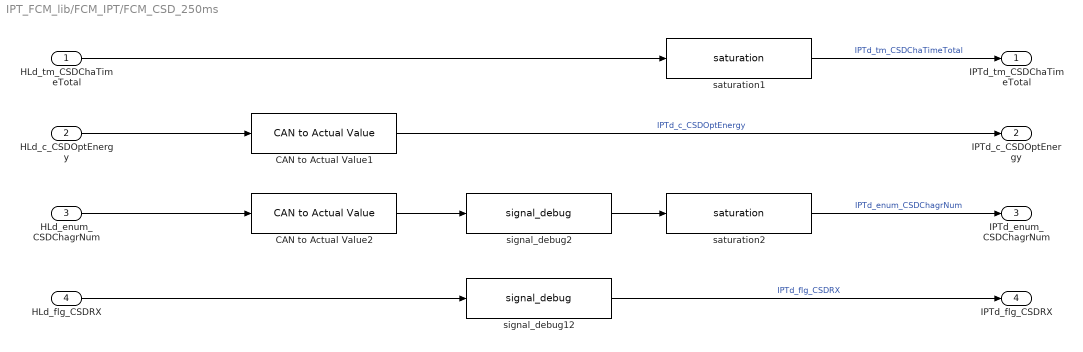
== system IPT_FCM_lib/FCM_IPT/FCM_CSD_250ms ==
  HLd_tm_CSDChaTimeTotal : Inport
  HLd_c_CSDOptEnergy : Inport  Port=2
  HLd_enum_CSDChagrNum : Inport  Port=3
  HLd_flg_CSDRX : Inport  Port=4
  CAN to Actual Value1 : Defined_Functionality/CAN to Actual Value  SystemSampleTime=-1  gain=0.1  offset=0
      settings: AttributesFormatString=[GAIN=%<gain>]\n[OFFSET=%<offset>]
  CAN to Actual Value2 : Defined_Functionality/CAN to Actual Value  SystemSampleTime=-1  gain=1  offset=1
      settings: AttributesFormatString=[GAIN=%<gain>]\n[OFFSET=%<offset>]
  saturation1 : Defined_Functionality/saturation  SystemSampleTime=-1  upper_limit=600  lower_limit=0
      settings: AttributesFormatString=[UPPER_LIMIT=%<upper_limit>]\n[LOWER_LIMIT=%<lower_limit>]
  saturation2 : Defined_Functionality/saturation  SystemSampleTime=-1  upper_limit=100  lower_limit=0
      settings: AttributesFormatString=[UPPER_LIMIT=%<upper_limit>]\n[LOWER_LIMIT=%<lower_limit>]
  signal_debug12 : Defined_Functionality/signal_debug  SystemSampleTime=-1  debug_switch=IPTc_dbgsw_CSDRX  debug_value=IPTc_dbgval_CSDRX
      settings: AttributesFormatString=[SWITCH=%<debug_switch>]\n[VALUE=%<debug_value>]
  signal_debug2 : Defined_Functionality/signal_debug  SystemSampleTime=-1  debug_switch=IPTc_dbgsw_CSDChagrNum  debug_value=IPTc_dbgval_CSDChagrNum
      settings: AttributesFormatString=[SWITCH=%<debug_switch>]\n[VALUE=%<debug_value>]
  IPTd_tm_CSDChaTimeTotal : Outport
  IPTd_c_CSDOptEnergy : Outport  Port=2
  IPTd_enum_CSDChagrNum : Outport  Port=3
  IPTd_flg_CSDRX : Outport  Port=4
  wires:
  HLd_flg_CSDRX/1 -> signal_debug12/1
  signal_debug12/1 -> IPTd_flg_CSDRX/1  "IPTd_flg_CSDRX"
  saturation2/1 -> IPTd_enum_CSDChagrNum/1  "IPTd_enum_CSDChagrNum"
  CAN to Actual Value1/1 -> IPTd_c_CSDOptEnergy/1  "IPTd_c_CSDOptEnergy"
  signal_debug2/1 -> saturation2/1
  saturation1/1 -> IPTd_tm_CSDChaTimeTotal/1  "IPTd_tm_CSDChaTimeTotal"
  CAN to Actual Value2/1 -> signal_debug2/1
  HLd_tm_CSDChaTimeTotal/1 -> saturation1/1
  HLd_enum_CSDChagrNum/1 -> CAN to Actual Value2/1
  HLd_c_CSDOptEnergy/1 -> CAN to Actual Value1/1

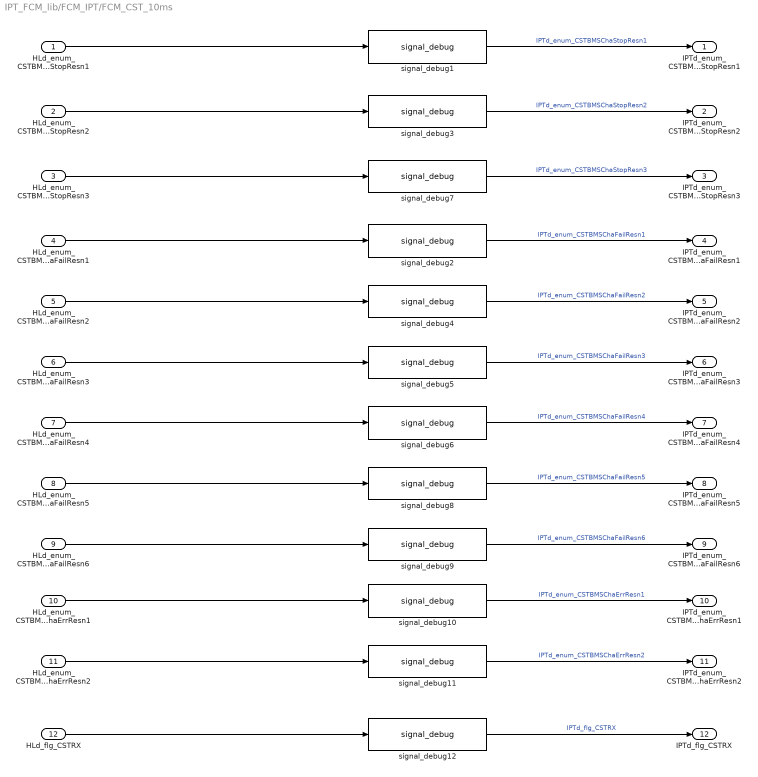
== system IPT_FCM_lib/FCM_IPT/FCM_CST_10ms ==
  HLd_enum_CSTBMSChaStopResn1 : Inport
  HLd_enum_CSTBMSChaStopResn2 : Inport  Port=2
  HLd_enum_CSTBMSChaStopResn3 : Inport  Port=3
  HLd_enum_CSTBMSChaFailResn1 : Inport  Port=4
  HLd_enum_CSTBMSChaFailResn2 : Inport  Port=5
  HLd_enum_CSTBMSChaFailResn3 : Inport  Port=6
  HLd_enum_CSTBMSChaFailResn4 : Inport  Port=7
  HLd_enum_CSTBMSChaFailResn5 : Inport  Port=8
  HLd_enum_CSTBMSChaFailResn6 : Inport  Port=9
  HLd_enum_CSTBMSChaErrResn1 : Inport  Port=10
  HLd_enum_CSTBMSChaErrResn2 : Inport  Port=11
  HLd_flg_CSTRX : Inport  Port=12
  signal_debug1 : Defined_Functionality/signal_debug  SystemSampleTime=-1  debug_switch=IPTc_dbgsw_CSTBMSChaStopResn1  debug_value=IPTc_dbgval_CSTBMSChaStopResn1
      settings: AttributesFormatString=[SWITCH=%<debug_switch>]\n[VALUE=%<debug_value>]
  signal_debug10 : Defined_Functionality/signal_debug  SystemSampleTime=-1  debug_switch=IPTc_dbgsw_CSTBMSChaErrResn1  debug_value=IPTc_dbgval_CSTBMSChaErrResn1
      settings: AttributesFormatString=[SWITCH=%<debug_switch>]\n[VALUE=%<debug_value>]
  signal_debug11 : Defined_Functionality/signal_debug  SystemSampleTime=-1  debug_switch=IPTc_dbgsw_CSTBMSChaErrResn2  debug_value=IPTc_dbgval_CSTBMSChaErrResn2
      settings: AttributesFormatString=[SWITCH=%<debug_switch>]\n[VALUE=%<debug_value>]
  signal_debug12 : Defined_Functionality/signal_debug  SystemSampleTime=-1  debug_switch=IPTc_dbgsw_CSTRX  debug_value=IPTc_dbgval_CSTRX
      settings: AttributesFormatString=[SWITCH=%<debug_switch>]\n[VALUE=%<debug_value>]
  signal_debug2 : Defined_Functionality/signal_debug  SystemSampleTime=-1  debug_switch=IPTc_dbgsw_CSTBMSChaFailResn1  debug_value=IPTc_dbgval_CSTBMSChaFailResn1
      settings: AttributesFormatString=[SWITCH=%<debug_switch>]\n[VALUE=%<debug_value>]
  signal_debug3 : Defined_Functionality/signal_debug  SystemSampleTime=-1  debug_switch=IPTc_dbgsw_CSTBMSChaStopResn2  debug_value=IPTc_dbgval_CSTBMSChaStopResn2
      settings: AttributesFormatString=[SWITCH=%<debug_switch>]\n[VALUE=%<debug_value>]
  signal_debug4 : Defined_Functionality/signal_debug  SystemSampleTime=-1  debug_switch=IPTc_dbgsw_CSTBMSChaFailResn2  debug_value=IPTc_dbgval_CSTBMSChaFailResn2
      settings: AttributesFormatString=[SWITCH=%<debug_switch>]\n[VALUE=%<debug_value>]
  signal_debug5 : Defined_Functionality/signal_debug  SystemSampleTime=-1  debug_switch=IPTc_dbgsw_CSTBMSChaFailResn3  debug_value=IPTc_dbgval_CSTBMSChaFailResn3
      settings: AttributesFormatString=[SWITCH=%<debug_switch>]\n[VALUE=%<debug_value>]
  signal_debug6 : Defined_Functionality/signal_debug  SystemSampleTime=-1  debug_switch=IPTc_dbgsw_CSTBMSChaFailResn4  debug_value=IPTc_dbgval_CSTBMSChaFailResn4
      settings: AttributesFormatString=[SWITCH=%<debug_switch>]\n[VALUE=%<debug_value>]
  signal_debug7 : Defined_Functionality/signal_debug  SystemSampleTime=-1  debug_switch=IPTc_dbgsw_CSTBMSChaStopResn3  debug_value=IPTc_dbgval_CSTBMSChaStopResn3
      settings: AttributesFormatString=[SWITCH=%<debug_switch>]\n[VALUE=%<debug_value>]
  signal_debug8 : Defined_Functionality/signal_debug  SystemSampleTime=-1  debug_switch=IPTc_dbgsw_CSTBMSChaFailResn5  debug_value=IPTc_dbgval_CSTBMSChaFailResn5
      settings: AttributesFormatString=[SWITCH=%<debug_switch>]\n[VALUE=%<debug_value>]
  signal_debug9 : Defined_Functionality/signal_debug  SystemSampleTime=-1  debug_switch=IPTc_dbgsw_CSTBMSChaFailResn6  debug_value=IPTc_dbgval_CSTBMSChaFailResn6
      settings: AttributesFormatString=[SWITCH=%<debug_switch>]\n[VALUE=%<debug_value>]
  IPTd_enum_CSTBMSChaStopResn1 : Outport
  IPTd_enum_CSTBMSChaStopResn2 : Outport  Port=2
  IPTd_enum_CSTBMSChaStopResn3 : Outport  Port=3
  IPTd_enum_CSTBMSChaFailResn1 : Outport  Port=4
  IPTd_enum_CSTBMSChaFailResn2 : Outport  Port=5
  IPTd_enum_CSTBMSChaFailResn3 : Outport  Port=6
  IPTd_enum_CSTBMSChaFailResn4 : Outport  Port=7
  IPTd_enum_CSTBMSChaFailResn5 : Outport  Port=8
  IPTd_enum_CSTBMSChaFailResn6 : Outport  Port=9
  IPTd_enum_CSTBMSChaErrResn1 : Outport  Port=10
  IPTd_enum_CSTBMSChaErrResn2 : Outport  Port=11  DataType=uint8  OutDataTypeStr=uint8
  IPTd_flg_CSTRX : Outport  Port=12
  wires:
  HLd_flg_CSTRX/1 -> signal_debug12/1
  signal_debug12/1 -> IPTd_flg_CSTRX/1  "IPTd_flg_CSTRX"
  HLd_enum_CSTBMSChaErrResn2/1 -> signal_debug11/1
  signal_debug11/1 -> IPTd_enum_CSTBMSChaErrResn2/1  "IPTd_enum_CSTBMSChaErrResn2"
  HLd_enum_CSTBMSChaErrResn1/1 -> signal_debug10/1
  signal_debug10/1 -> IPTd_enum_CSTBMSChaErrResn1/1  "IPTd_enum_CSTBMSChaErrResn1"
  signal_debug9/1 -> IPTd_enum_CSTBMSChaFailResn6/1  "IPTd_enum_CSTBMSChaFailResn6"
  signal_debug8/1 -> IPTd_enum_CSTBMSChaFailResn5/1  "IPTd_enum_CSTBMSChaFailResn5"
  signal_debug6/1 -> IPTd_enum_CSTBMSChaFailResn4/1  "IPTd_enum_CSTBMSChaFailResn4"
  signal_debug5/1 -> IPTd_enum_CSTBMSChaFailResn3/1  "IPTd_enum_CSTBMSChaFailResn3"
  signal_debug4/1 -> IPTd_enum_CSTBMSChaFailResn2/1  "IPTd_enum_CSTBMSChaFailResn2"
  signal_debug2/1 -> IPTd_enum_CSTBMSChaFailResn1/1  "IPTd_enum_CSTBMSChaFailResn1"
  HLd_enum_CSTBMSChaFailResn6/1 -> signal_debug9/1
  HLd_enum_CSTBMSChaFailResn5/1 -> signal_debug8/1
  HLd_enum_CSTBMSChaFailResn4/1 -> signal_debug6/1
  HLd_enum_CSTBMSChaFailResn3/1 -> signal_debug5/1
  HLd_enum_CSTBMSChaFailResn2/1 -> signal_debug4/1
  HLd_enum_CSTBMSChaFailResn1/1 -> signal_debug2/1
  signal_debug7/1 -> IPTd_enum_CSTBMSChaStopResn3/1  "IPTd_enum_CSTBMSChaStopResn3"
  signal_debug3/1 -> IPTd_enum_CSTBMSChaStopResn2/1  "IPTd_enum_CSTBMSChaStopResn2"
  HLd_enum_CSTBMSChaStopResn3/1 -> signal_debug7/1
  HLd_enum_CSTBMSChaStopResn2/1 -> signal_debug3/1
  HLd_enum_CSTBMSChaStopResn1/1 -> signal_debug1/1
  signal_debug1/1 -> IPTd_enum_CSTBMSChaStopResn1/1  "IPTd_enum_CSTBMSChaStopResn1"

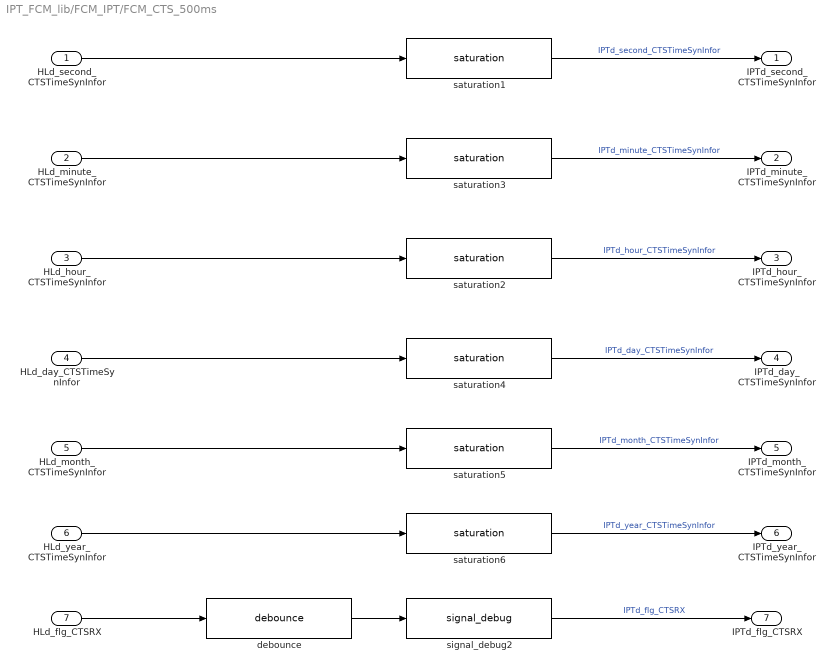
== system IPT_FCM_lib/FCM_IPT/FCM_CTS_500ms ==
  HLd_second_CTSTimeSynInfor : Inport
  HLd_minute_CTSTimeSynInfor : Inport  Port=2
  HLd_hour_CTSTimeSynInfor : Inport  Port=3
  HLd_day_CTSTimeSynInfor : Inport  Port=4
  HLd_month_CTSTimeSynInfor : Inport  Port=5
  HLd_year_CTSTimeSynInfor : Inport  Port=6
  HLd_flg_CTSRX : Inport  Port=7
  debounce : Defined_Functionality/debounce  SystemSampleTime=-1  debounce_time=30
      settings: AttributesFormatString=[DEBOUNCE_TIME=%<debounce_time>]
  saturation1 : Defined_Functionality/saturation  SystemSampleTime=-1  upper_limit=60  lower_limit=0
      settings: AttributesFormatString=[UPPER_LIMIT=%<upper_limit>]\n[LOWER_LIMIT=%<lower_limit>]
  saturation2 : Defined_Functionality/saturation  SystemSampleTime=-1  upper_limit=24  lower_limit=0
      settings: AttributesFormatString=[UPPER_LIMIT=%<upper_limit>]\n[LOWER_LIMIT=%<lower_limit>]
  saturation3 : Defined_Functionality/saturation  SystemSampleTime=-1  upper_limit=60  lower_limit=0
      settings: AttributesFormatString=[UPPER_LIMIT=%<upper_limit>]\n[LOWER_LIMIT=%<lower_limit>]
  saturation4 : Defined_Functionality/saturation  SystemSampleTime=-1  upper_limit=31  lower_limit=0
      settings: AttributesFormatString=[UPPER_LIMIT=%<upper_limit>]\n[LOWER_LIMIT=%<lower_limit>]
  saturation5 : Defined_Functionality/saturation  SystemSampleTime=-1  upper_limit=12  lower_limit=0
      settings: AttributesFormatString=[UPPER_LIMIT=%<upper_limit>]\n[LOWER_LIMIT=%<lower_limit>]
  saturation6 : Defined_Functionality/saturation  SystemSampleTime=-1  upper_limit=2235  lower_limit=1985
      settings: AttributesFormatString=[UPPER_LIMIT=%<upper_limit>]\n[LOWER_LIMIT=%<lower_limit>]
  signal_debug2 : Defined_Functionality/signal_debug  SystemSampleTime=-1  debug_switch=IPTc_dbgsw_CTSRX  debug_value=IPTc_dbgval_CTSRX
      settings: AttributesFormatString=[SWITCH=%<debug_switch>]\n[VALUE=%<debug_value>]
  IPTd_second_CTSTimeSynInfor : Outport
  IPTd_minute_CTSTimeSynInfor : Outport  Port=2
  IPTd_hour_CTSTimeSynInfor : Outport  Port=3
  IPTd_day_CTSTimeSynInfor : Outport  Port=4
  IPTd_month_CTSTimeSynInfor : Outport  Port=5
  IPTd_year_CTSTimeSynInfor : Outport  Port=6
  IPTd_flg_CTSRX : Outport  Port=7
  wires:
  debounce/1 -> signal_debug2/1
  HLd_flg_CTSRX/1 -> debounce/1
  signal_debug2/1 -> IPTd_flg_CTSRX/1  "IPTd_flg_CTSRX"
  saturation6/1 -> IPTd_year_CTSTimeSynInfor/1  "IPTd_year_CTSTimeSynInfor"
  HLd_year_CTSTimeSynInfor/1 -> saturation6/1
  saturation4/1 -> IPTd_day_CTSTimeSynInfor/1  "IPTd_day_CTSTimeSynInfor"
  saturation5/1 -> IPTd_month_CTSTimeSynInfor/1  "IPTd_month_CTSTimeSynInfor"
  HLd_month_CTSTimeSynInfor/1 -> saturation5/1
  HLd_day_CTSTimeSynInfor/1 -> saturation4/1
  saturation2/1 -> IPTd_hour_CTSTimeSynInfor/1  "IPTd_hour_CTSTimeSynInfor"
  HLd_hour_CTSTimeSynInfor/1 -> saturation2/1
  saturation3/1 -> IPTd_minute_CTSTimeSynInfor/1  "IPTd_minute_CTSTimeSynInfor"
  HLd_minute_CTSTimeSynInfor/1 -> saturation3/1
  saturation1/1 -> IPTd_second_CTSTimeSynInfor/1  "IPTd_second_CTSTimeSynInfor"
  HLd_second_CTSTimeSynInfor/1 -> saturation1/1
